simulink model "rctMultiUncertainModel"  (R2023a)
settings: Solver=ode45  StartTime=0.0  StopTime=10.0  RelTol=1e-3  EnableMultiTasking=on
PreLoadFcn:
  | input_unc = ultidyn('input_unc',[1 1]);
  | wt = makeweight(0.25,130,2.5);
  | unc_sys = ss(ureal('a',-1,'Range',[-2 -.5]),1,5,0);
  | vals = [];
libraries: RCTblocks x3
settings Model: Creator=The MathWorks, Inc.  LastModifiedBy=The MathWorks, Inc.
settings SolverCC: AlgebraicLoopSolver=TrustRegion
settings DataIOCC: LimitDataPoints=on  SaveFormat=Array  ReturnWorkspaceOutputs=off
settings OptimizationCC: ExpressionDepthLimit=2147483647  LifeSpan=inf
settings DebuggingCC: UnderspecifiedInitializationDetection=Classic  MergeDetectMultiDrivingBlocksExec=none  FcnCallInpInsideContextMsg=warning  UnconnectedInputMsg=warning  UnconnectedOutputMsg=warning  UnconnectedLineMsg=warning  StateNameClashWarn=warning  SFUnexpectedBacktrackingDiag=warning  SFNoUnconditionalDefaultTransitionDiag=warning  SFExecutionAtInitializationDiag=none  ArithmeticOperatorsInVariantConditions=warning
settings HardwareCC: ProdBitPerPointer=32  ProdBitPerSizeT=32  ProdBitPerPtrDiffT=32  ProdLargestAtomicFloat=None  ProdIntDivRoundTo=Undefined  ProdEndianess=Unspecified  ProdWordSize=32  ProdHWDeviceType=32-bit Generic
settings ModelReferenceCC: EnableRefExpFcnMdlSchedulingChecks=on  PropagateSignalLabelsOutOfModel=off
settings SFSimCC: SimUseLocalCustomCode=off  CustomCodeUndefinedFunction=UseInterfaceOnly
settings RTWCC: RTWUseLocalCustomCode=off  DLArmComputeVersion=19.05
settings CodeAppCC: StateflowObjectComments=on
settings GRTTargetCC: TargetLangStandard=C89/C90 (ANSI)  CombineOutputUpdateFcns=off  GRTInterface=on
settings ConfigComp: CovMetricSettings=dw  CovSaveCumulativeToWorkspaceVar=on  CovSaveSingleToWorkspaceVar=on  CovExternalEMLEnable=off

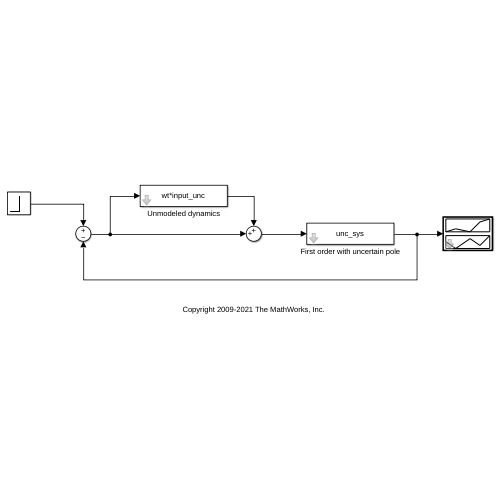
[thumbnail: Simulink's stored preview of the top-level diagram]
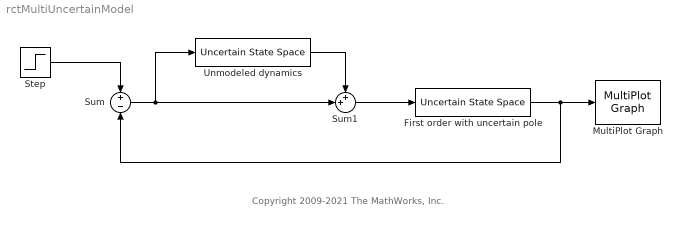
== system rctMultiUncertainModel ==
  note: Copyright 2009-2021 The MathWorks, Inc.
  First order with uncertain pole : RCTblocks/Uncertain State Space  Tag=USS  USystem=unc_sys  UValue=vals  X0=[]  uX0=[]
  MultiPlot Graph : RCTblocks/MultiPlot Graph  Tag=MultiPlot  tmin=0  tmax=5  ymin=-0.5  ymax=1.5  vnamesave=multisimout
  Step : Step  SampleTime=0
  Sum : Sum  Inputs=+-
  Sum1 : Sum  Inputs=++|
  Unmodeled dynamics : RCTblocks/Uncertain State Space  Tag=USS  USystem=wt*input_unc  UValue=vals  X0=[]  uX0=[]
  wires:
  Unmodeled dynamics/1 -> Sum1/1
  Sum1/1 -> First order with uncertain pole/1
  First order with uncertain pole/1 -> MultiPlot Graph/1, Sum/2
  Sum/1 -> Sum1/2, Unmodeled dynamics/1
  Step/1 -> Sum/1
